simulink model "ex4_8a"  (R2020b)
settings: Solver=VariableStepAuto  StartTime=0.0  StopTime=4.096  RelTol=1e-3
settings Model: Creator=seojoon  LastModifiedBy=seojoon

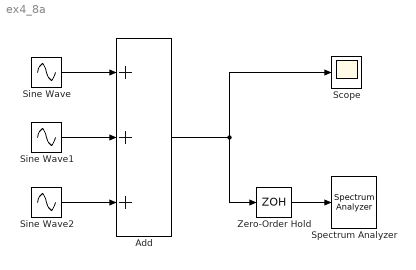
== system ex4_8a ==
  Add : Sum  Inputs=+++
  Scope : Scope
  Sine Wave : Sin  Amplitude=10  Frequency=2*pi*50  SampleTime=0
  Sine Wave1 : Sin  Amplitude=10  Frequency=2*pi*100  Phase=pi/2  SampleTime=0
  Sine Wave2 : Sin  Amplitude=-10  Frequency=2*pi*200  SampleTime=0
  Spectrum Analyzer : SpectrumAnalyzer
  Zero-Order Hold : ZeroOrderHold  SampleTime=1e-3
  wires:
  Sine Wave/1 -> Add/1
  Sine Wave1/1 -> Add/2
  Sine Wave2/1 -> Add/3
  Add/1 -> Scope/1, Zero-Order Hold/1
  Zero-Order Hold/1 -> Spectrum Analyzer/1
